simulink model "TrayectoriaObstaculos"  (R2023b)
settings: Solver=FixedStepAuto  StartTime=0.0  StopTime=300  RelTol=1e-3  EnableMultiTasking=on
model workspace (MAT data in the model file):
  d = 1
libraries: robotalgslib x1
settings Model: ExtModeTrigDuration=2  Creator=Usuario_UMA  LastModifiedBy=Daniel
settings OptimizationCC: EnhancedBackFolding=on  PassReuseOutputArgsAs=Individual arguments  ZeroExternalMemoryAtStartup=off  ZeroInternalMemoryAtStartup=off  MaxStackSize=64  OptimizeBlockOrder=speed  DifferentSizesBufferReuse=on  EfficientTunableParamExpr=on
settings DebuggingCC: ParameterTunabilityLossMsg=error
settings HardwareCC: ProdBitPerInt=16  ProdBitPerPointer=16  ProdBitPerSizeT=16  ProdBitPerPtrDiffT=16  ProdLargestAtomicFloat=None  ProdWordSize=8  ProdHWDeviceType=Atmel->AVR
settings SFSimCC: MATLABDynamicMemAlloc=off
settings RTWCC: Description=Embedded Coder  SystemTargetFile=ert.tlc  HardwareBoard=Arduino Mega 2560  TemplateMakefile=ert_default_tmf  Toolchain=Arduino AVR  BuildConfiguration=Faster Runs
settings CodeAppCC: ForceParamTrailComments=on  IgnoreCustomStorageClasses=off  OperatorAnnotations=on  SimulinkDataObjDesc=on  SFDataObjDesc=on  InsertBlockDesc=on
settings ERTTargetCC: SupportContinuousTime=on  SupportVariableSizeSignals=on  ExtModeTransport=3  ExtModeStaticAlloc=on  ExtModeAutomaticAllocSize=off  ExtModeStaticAllocSize=2048  ExtModeMexFile=ext_xcp  ExtModeIntrfLevel=Level2 - Open

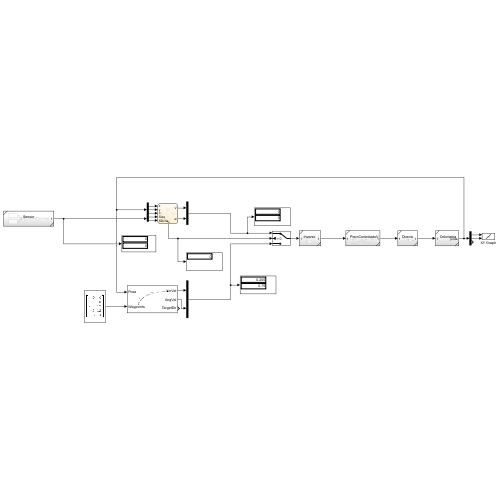
[thumbnail: Simulink's stored preview of the top-level diagram]
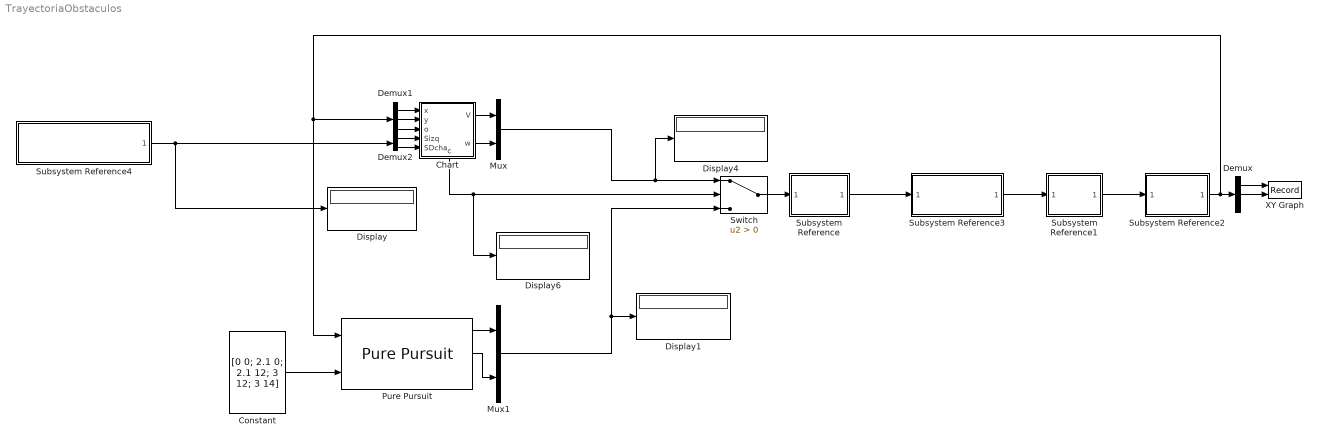
== system TrayectoriaObstaculos ==
  Chart : Stateflow chart  TreatAsAtomicUnit=on
      settings: PortSchema="{\"entries\":[{\"content\":{\"sides\":[{\"content\":{\"connectorIds\":[\"In1\",\"In2\",\"In3\",\"In4\",\"In5\"]},\"type\":\"ConnectorPlacement.EquallySpacedRectSide\",\"uuid\":\"0c906aa7-8786-49a2-ba1f-534800ed0484\"},{\"content\":{\"connectorIds\":[\"Out2\",\"Out3\"],\"side\":\"RIGHT\"},\"type\":\"ConnectorPlacement.EquallySpacedRectSide\",\"uuid\":\"f74849c7-163d-4f95-977c-475817888a5e\"},{\"content\":{\"side\":\"TOP\"},\"type\":\"ConnectorPlacement.EquallySpacedRectSide\",\"uuid\":\"137f602b-afd6-4481-a0e3-0dc845197e96\"},{\"content\":{\"connectorIds\":[\"Out1\"],\"side\":\"BOTTOM\"},\"type\":\"ConnectorPlacement.EquallySpacedRectSide\",\"uuid\":\"f9e4e3a7-68ad-4ed3-96eb-a456541ca525\"}]},\"type\":\"ConnectorPlacement.EquallySpacedConnector\",\"uuid\":\"c72bb38c-8788-4f09-8069-2512b987828d\"}],\"packageUris\":[\"http://schema.mathworks.com/mf0/Connector/R2020b\"],\"version\":\"1.0\"}"
  Constant : Constant  Value=[0 0; 2.1 0; 2.1 12; 3 12; 3 14]
  Demux : Demux  Outputs=3
  Demux1 : Demux  Outputs=3
  Demux2 : Demux  Outputs=2
  Display{,1,4,6} (4 alike) : Display
  Mux : Mux  Inputs=2
  Mux1 : Mux  Inputs=2
  Pure Pursuit : robotalgslib/Pure Pursuit  DesiredLinearVelocity=0.205  MaxAngularVelocity=0.75  LookaheadDistance=0.3  TargetDirPort=on  SimulateUsing=Interpreted execution
      settings: LibrarySourceBlock=navlib/Control Algorithms/Pure Pursuit
  Subsystem Reference : Subsystem  ReferencedSubsystem=Inverso
  Subsystem Reference1 : Subsystem  ReferencedSubsystem=Directo
  Subsystem Reference2 : Subsystem  ReferencedSubsystem=Odometria
  Subsystem Reference3 : Subsystem  ReferencedSubsystem=PieroControladoV
  Subsystem Reference4 : Subsystem  ReferencedSubsystem=Sensor
  Switch : Switch  Criteria=u2 > Threshold  SaturateOnIntegerOverflow=off  InputSameDT=off
  XY Graph : Record  FileSettingsInternal="{\"entries\":[{\"content\":{\"excelSettings\":{\"content\":{},\"type\":\"Streamout.ExcelSettings\"}},\"type\":\"Streamout.FileSettingStorage\",\"uuid\":\"\"}],\"packageUris\":[\"http:\\/\\/schema.mathworks.com\\/mf0\\/streamout_blocks\\/R2020a\"],\"version\":\"1.0\"}"  Layout=[1 1]  SignalsInternal="{\"entries\":[{\"content\":{\"signals\":[{\"content\":{\"blockPath\":[],\"dimensions\":[1],\"domain\":\"\",\"lineColor\":\"#0072bd\",\"plots\":[ 1 ],\"port\":1,\"sid\":[\"\"],\"signalID\":1,\"signalName\":\"Demux:1\"},\"type\":\"RecordBlkView.Signal\",\"uuid\":\"\"},{\"content\":{\"blockPath\":[],\"dimensions\":[1],\"domain\":\"\",\"lineColor\":\"#d95319\",\"plots\":[ 1 ],\"port\":2,\"sid\":[\"\"],\"signalID\":2,\"signalName\":\"Demux:2\"},\"type\":\"RecordBlkView.Signal\",\"uuid\":\"\"}]},\"type\":\"RecordBlkView.InputSignals\",\"uuid\":\"\"}],\"packageUris\":[\"http:\\/\\/schema.mathworks.com\\/mf0\\/streamout_blocks\\/R2020a\"],\"version\":\"1.0\"}"  VisualizationBindings="{\"xyplotplugin\":{\"info\":[{\"series\":[{\"bindingParametersList\":[{\"parameter\":\"X-Axis\",\"signalID\":1,\"signalName\":\"Demux:1\"},{\"parameter\":\"Y-Axis\",\"signalID\":2,\"signalName\":\"Demux:2\"}],\"seriesID\":0}],\"subplotID\":1}]}}"  CompatibilityTag=XY
  wires:
  Subsystem Reference/1 -> Subsystem Reference3/1
  Subsystem Reference3/1 -> Subsystem Reference1/1
  Subsystem Reference1/1 -> Subsystem Reference2/1
  Subsystem Reference2/1 -> Pure Pursuit/1, Demux1/1, Demux/1
  Demux/2 -> XY Graph/2
  Demux/1 -> XY Graph/1
  Switch/1 -> Subsystem Reference/1
  Constant/1 -> Pure Pursuit/2
  Chart/3(w) -> Mux/2
  Chart/2(V) -> Mux/1
  Pure Pursuit/1 -> Mux1/1
  Mux1/1 -> Switch/3, Display1/1
  Mux/1 -> Display4/1, Switch/1
  Demux1/1 -> Chart/1(x)
  Demux1/2 -> Chart/2(y)
  Demux1/3 -> Chart/3(o)
  Chart/1(c) -> Switch/2, Display6/1
  Demux2/1 -> Chart/4(Sizq)
  Demux2/2 -> Chart/5(SDcha)
  Pure Pursuit/2 -> Mux1/2
  Subsystem Reference4/1 -> Demux2/1, Display/1

== stateflow chart TrayectoriaObstaculos/Chart ==
  state SinObstaculos
    w=0;
    V=0;
    c=0;
  state ObstaculosIzq
    w=-pi/4;
    V=0.1;
    c=1;
  state ObstaculosDcha
    w=pi/4;
    V=0.1;
    c=1;
  state ObstaculosFrente
    w=pi/2;
    V=0;
    c=1;
  (default) -> SinObstaculos
  SinObstaculos -> ObstaculosIzq : [Sizq<40]
  ObstaculosDcha -> SinObstaculos [order 1] : [SDcha<40]
  ObstaculosIzq -> SinObstaculos [order 2] : after(1,sec)
  ObstaculosFrente -> SinObstaculos [order 2] : after(1.5,sec)
  ObstaculosDcha -> SinObstaculos [order 2] : after(1,sec)
  ObstaculosIzq -> ObstaculosFrente [order 1] : [SDcha<40]
  ObstaculosFrente -> ObstaculosDcha [order 1] : [Sizq<40]
  data: c output; V output double size=1; w output double size=1; x input; y input; o input; Sizq input; SDcha input
